simulink model "BLDC_CurrentLoop"  (R2019b)
settings: Solver=FixedStepDiscrete  StartTime=0.0  StopTime=0.0025  FixedStep=Ts  MaxStep=Ts  RelTol=1e-3
values from neighbouring files (symbols this model uses):
  C_1 = B_0/A_0    (= 1.99999600001e-06)    [SetupSimulation.m]
  C_2 = B_1/A_0    (= 1.99999600001e-06)    [SetupSimulation.m]
  count_max = 500-1    (= 499)    [SetupSimulation.m]
  D_1 = A_1/A_0    (= -0.999996000008)    [SetupSimulation.m]
  test_bemf = 1    [SetupSimulation.m]
  Vsupply = 12    [SetupSimulation.m]
libraries: simulink x1
settings Model: Creator=rahuliyer  LastModifiedBy=rahuliyer
settings DebuggingCC: ParameterOverflowMsg=warning

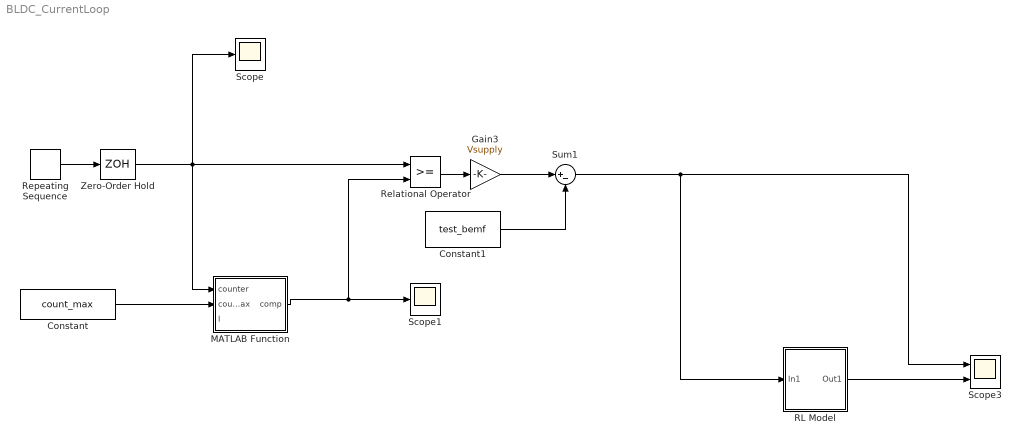
== system BLDC_CurrentLoop ==
  Constant : Constant  Value=count_max  OutDataTypeStr=Inherit: Inherit via back propagation  SampleTime=-1
  Constant1 : Constant  Value=test_bemf
  Gain3 : Gain  Gain=Vsupply
  MATLAB Function : MATLAB Function  TreatAsAtomicUnit=on
  RL Model : Subsystem
  Relational Operator : RelationalOperator  OutDataTypeStr=boolean  RndMeth=Simplest
  Repeating Sequence : simulink/Sources/Repeating Sequence  rep_seq_t=triangle_times  rep_seq_y=triangle_vals
  Scope : Scope
  Scope1 : Scope
  Scope3 : Scope  NumInputPorts=2
  Sum1 : Sum  Inputs=|+-
  Zero-Order Hold : ZeroOrderHold  SampleTime=-1
  wires:
  MATLAB Function/1(comp) -> Scope1/1, Relational Operator/2
  Constant/1 -> MATLAB Function/2(count_max)
  Repeating Sequence/1 -> Zero-Order Hold/1
  Zero-Order Hold/1 -> MATLAB Function/1(counter), Scope/1, Relational Operator/1
  Relational Operator/1 -> Gain3/1
  Gain3/1 -> Sum1/1
  Constant1/1 -> Sum1/2
  Sum1/1 -> Scope3/1, RL Model/1(In1)
  RL Model/1(Out1) -> Scope3/2

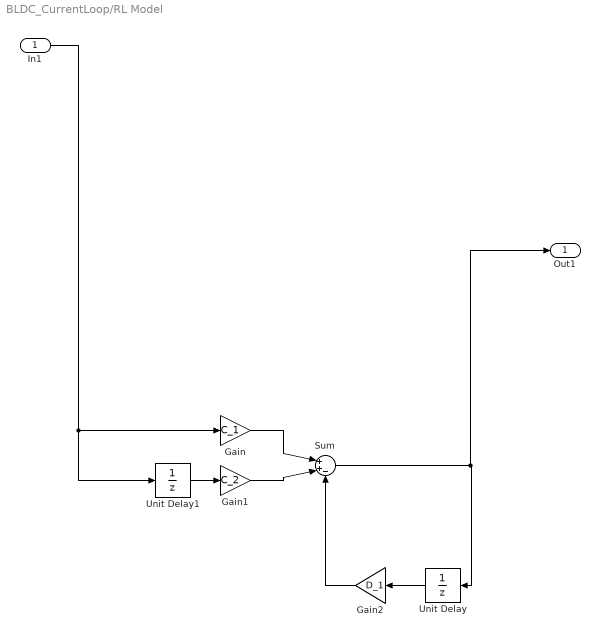
== system BLDC_CurrentLoop/RL Model ==
  In1 : Inport
  Gain : Gain  Gain=C_1  OutDataTypeStr=double
  Gain1 : Gain  Gain=C_2  OutDataTypeStr=double
  Gain2 : Gain  Gain=D_1  OutDataTypeStr=double
  Sum : Sum  Inputs=|++-
  Unit Delay : UnitDelay  SampleTime=-1  HasFrameUpgradeWarning=on
  Unit Delay1 : UnitDelay  SampleTime=-1  HasFrameUpgradeWarning=on
  Out1 : Outport
  wires:
  In1/1 -> Gain/1, Unit Delay1/1
  Unit Delay1/1 -> Gain1/1
  Unit Delay/1 -> Gain2/1
  Gain2/1 -> Sum/3
  Sum/1 -> Out1/1, Unit Delay/1
  Gain1/1 -> Sum/2
  Gain/1 -> Sum/1

== matlab function BLDC_CurrentLoop/MATLAB Function ==
  data: counter input; comp output; count_max input; I input
function comp = fcn(counter,count_max,I)
persistent compareval
if isempty(compareval)
    compareval = count_max;
end
if (counter == count_max)
    % sample current and do PI control
    compareval = 415;
end

comp = compareval;
